simulink model "puntoc_simulink_200901"  (R2019a)
settings: Solver=VariableStepAuto  StartTime=0.0  StopTime=20.0  RelTol=1e-3
values from neighbouring files (symbols this model uses):
  ingresso = 10    [puntoc_200901.m]
  R = 5    [puntoc_200901.m]
libraries: cstblocks x1
settings Model: Creator=Marco Greco  LastModifiedBy=Marco Greco

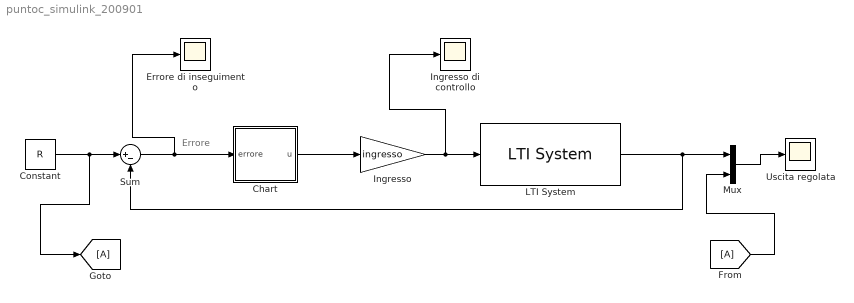
== system puntoc_simulink_200901 ==
  note: Errore
  Chart : Stateflow chart  BlockKeywords=__PRM__SERIALIZED__DATA__:Stateflow Chart,Stateflow Diagram  TreatAsAtomicUnit=on
  Constant : Constant  Value=R
  "Errore di inseguimento " : Scope
  Ingresso : Gain  Gain=ingresso
  Ingresso di controllo : Scope
  LTI System : cstblocks/LTI System  sys=G  IC=[]
  Mux : Mux  Inputs=2
  Sum : Sum  Inputs=|+-
  Uscita regolata : Scope
  wires:
  Constant/1 -> [A], Sum/1
  Sum/1 -> "Errore di inseguimento "/1, Chart/1(errore)
  Chart/1(u) -> Ingresso/1
  Ingresso/1 -> Ingresso di controllo/1, LTI System/1
  LTI System/1 -> Sum/2, Mux/1
  [A] -> Mux/2
  Mux/1 -> Uscita regolata/1

== stateflow chart puntoc_simulink_200901/Chart ==
  settings: updateMethod=CONTINUOUS
  state ON
    entry:
    u=1;
  state OFF
    entry:
    u=0;
  (default) -> ON
  OFF -> ON : [errore >= epsilon]
  ON -> OFF : [errore <= -epsilon]
  data: epsilon parameter; errore input; u output
